simulink model "ecdraw"  (R2015a)
settings: Solver=ode45  StartTime=0.0  StopTime=10.0  RelTol=1e-3
settings Model: Creator=asus  LastModifiedBy=asus

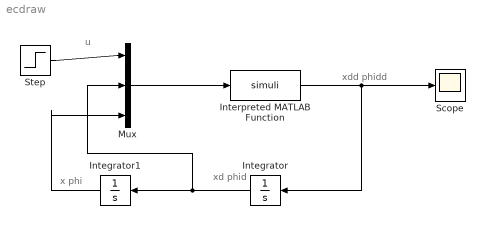
== system ecdraw ==
  note: x phi
  note: xd phid
  note: xdd phidd
  note: u
  Integrator : Integrator  InitialCondition=[0;0]
  Integrator1 : Integrator  InitialCondition=[.1 30*pi/180]'
  Interpreted MATLAB Function : MATLABFcn  MATLABFcn=simuli
  Mux : Mux  Inputs=3
  Scope : Scope
  Step : Step  SampleTime=0
  wires:
  Mux/1 -> Interpreted MATLAB Function/1
  Interpreted MATLAB Function/1 -> Scope/1, Integrator/1
  Integrator/1 -> Mux/2, Integrator1/1
  Step/1 -> Mux/1
  Integrator1/1 -> Mux/3
